simulink model "CubeSatModel_pert"  (R2024a)
settings: Solver=FixedStepAuto  StartTime=0.0  StopTime=5467.6512  FixedStep=0.5  MaxStep=10  RelTol=1e-6  AbsTol=1e-7
undefined symbols (not defined in the file): juliandate
libraries: aerolibutil x12, aerolibconvert2 x4, slpidlib x1, sharedtransform x1, aerolibsatdyn x1, aerolibobsolete x1, aerolibattitudesys x1, simulink x1, vrlib x1
settings Model: Creator=The MathWorks, Inc.  LastModifiedBy=sandr
settings SolverCC: MaxConsecutiveMinStep=10  AutoInsertRateTranBlk=on  DecoupledContinuousIntegration=on  MinimalZcImpactIntegration=on  MaxZcPerStep=1
settings DebuggingCC: ReadBeforeWriteMsg=DisableAll  WriteAfterWriteMsg=DisableAll  WriteAfterReadMsg=DisableAll  MultiTaskDSMMsg=none  UnconnectedInputMsg=warning  UnconnectedOutputMsg=warning  UnconnectedLineMsg=warning
settings ModelReferenceCC: UpdateModelReferenceTargets=IfOutOfDate  EnableRefExpFcnMdlSchedulingChecks=on
settings SFSimCC: SFSimEcho=off
settings RTWCC: GPUComputeCapability=3.5  DLArmComputeVersion=19.05

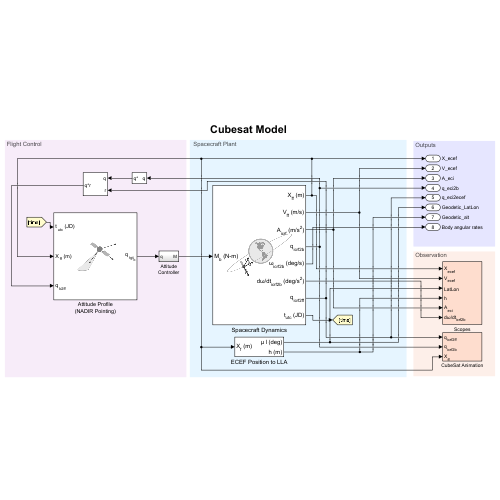
[thumbnail: Simulink's stored preview of the top-level diagram]
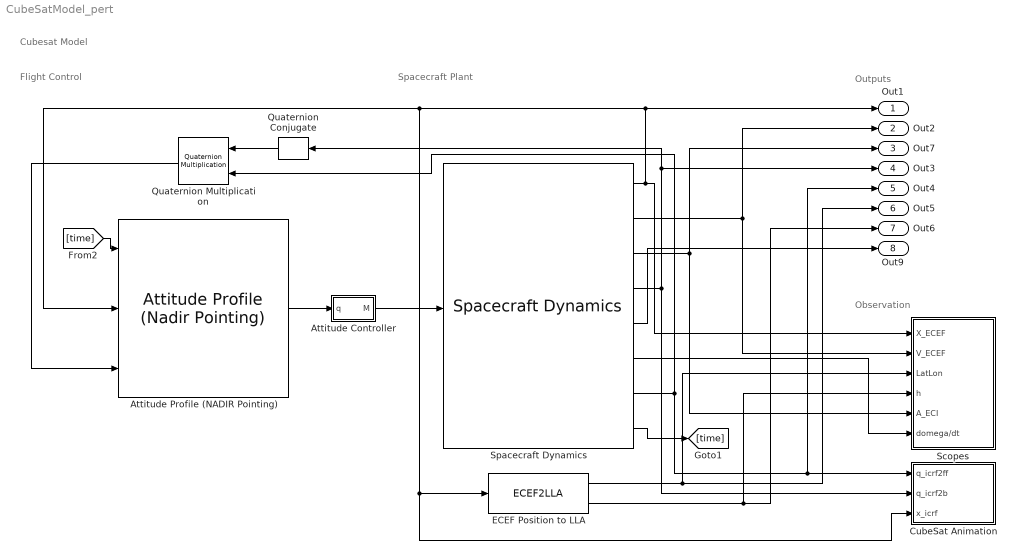
== system CubeSatModel_pert ==
  note: Flight Control
  note: Outputs
  note: Spacecraft Plant
  note: Observation
  note: Cubesat Model
  Attitude Controller : Subsystem
  Attitude Profile (NADIR Pointing) : aerolibsatdyn/Attitude Profile (Nadir Pointing)  outputError=on  outputFinalAttitude=off  portFrame=Fixed-frame  pointingMode=Point at nadir  celestialTarget=Sun  tunablePointing=off  primaryAlignmentSrc=Dialog  primaryAlignment=[0 0 1]  secondaryAlignmentSrc=Dialog  secondaryAlignment=[1 0 0]  constraintFrame=ICRF  primaryConstraintSrc=Dialog  primaryConstraint=[1 0 0]  secondaryConstraintSrc=Dialog  secondaryConstraint=[0 1 0]
  CubeSat Animation : Subsystem  mask(Simulink 3D Animation of CubeSat){enableVis=on, startDate=juliandate(2020, 1, 1, 12, 0, 0), visSampleTime=5, cubesatSize=2e5, showAntenna=on, antennaHeight=1e6, antennaHalfAngle=15}
      mask prompts: enableVis "spacecraft:cubesat:AnimEnableVis"; startDate "spacecraft:cubesat:StartDate"; visSampleTime "spacecraft:cubesat:AnimSampleTime"; cubesatSize "spacecraft:cubesat:MdlSize"; showAntenna "spacecraft:cubesat:ShowCone"; antennaHeight "spacecraft:cubesat:ConeHeight"; antennaHalfAngle "spacecraft:cubesat:ConeAngle"
      mask help: spacecraft:cubesat:VisBlockDesc
      settings: OpenFcn=|
      | if ~builtin('license','test','virtual_reality_toolbox')
      |     set_param(gcb, 'enableVis', 'off');
      | end
      | open_system(gcb,'mask');
      mask Callback enableVis:
      | if strcmp(get_param(gcb,'enableVis'), 'on')
      |     [licAvail, ~] = builtin('license','checkout','Virtual_Reality_Toolbox');
      |     if licAvail
      |         enable = repmat({'on'},7,1);
      |         set_param(gcb, 'Commented', 'off');
      |     else
      |         enable = repmat({'off'},7,1);
      |         set_param(gcb, 'Commented', 'on');
      |         set_param(gcb,'enableVis', 'off');
      |     end
      |     clear licAvail
      | else
      |     enable = repmat({'off'},7,1);
      |     set_param(gcb, 'Commented', 'on');
      | end
      | enable{1} = 'on';
      | set_param(gcb,'MaskEnables', enable);
      | clear enable
      mask Callback showAntenna:
      | if strcmp(get_param(gcb, 'enableVis'), 'on')
      |     enable = get_param(gcb,'MaskEnables');
      |     if strcmp(get_param(gcb, 'showAntenna'), 'off')
      |         enable(6:7) = {'off'};
      |     else
      |         enable(6:7) = {'on'};
      |     end
      |     set_param(gcb,'MaskEnables', enable);
      |     clear enable
      | end
      mask DialogControl enableVis Prompt: Enable visualization with Simulink 3D Animation
      mask DialogControl vrOpenBtn Prompt: spacecraft:cubesat:AnimOpenBtn
      mask DialogControl vrOpenBtn Callback:
      | if builtin('license','checkout','Virtual_Reality_Toolbox')
      |     vrmfunc('FnOpen',getSimulinkBlockHandle([gcb '/VR Sink']));
      | end
      mask DialogControl startDate Prompt: Start date [Julian date]:
      mask DialogControl startDate Tooltip: spacecraft:cubesat:StartDateTT
      mask DialogControl visSampleTime Prompt: Animation refresh rate:
      mask DialogControl visSampleTime Tooltip: spacecraft:cubesat:AnimSampleTimeTT
      mask DialogControl cubesatSize Prompt: CubeSat display size [m]:
      mask DialogControl cubesatSize Tooltip: spacecraft:cubesat:MdlSizeTT
      mask DialogControl Container3 Prompt: spacecraft:cubesat:AntennaPropArea
      mask DialogControl showAntenna Prompt: Show antenna cone in animation
      mask DialogControl showAntenna Tooltip: spacecraft:cubesat:ShowConeTT
      mask DialogControl antennaHeight Prompt: Antenna cone height [m]:
      mask DialogControl antennaHeight Tooltip: spacecraft:cubesat:ConeHeightTT
      mask DialogControl antennaHalfAngle Prompt: Antenna cone half angle [deg]:
      mask DialogControl antennaHalfAngle Tooltip: spacecraft:cubesat:ConeAngleTT
      mask Display:
      | port_label('input', 3, 'X_{ff}','texmode','on')
      | port_label('input', 2, 'q_{icrf2b}','texmode','on')
      | port_label('input', 1, 'q_{icrf2ff}','texmode','on')
  ECEF Position to LLA : ECEF2LLA  R=6378137
  Quaternion Conjugate : aerolibutil/Quaternion Conjugate
  Quaternion Multiplication : aerolibutil/Quaternion Multiplication
  Scopes : Subsystem  VariantControl=visOff
      mask Display:
      | port_label('input', 1, 'X_{ecef}','texmode','on')
      | port_label('input', 2, 'V_{ecef}','texmode','on')
      | port_label('input', 3, 'LatLon','texmode','on')
      | port_label('input', 4, 'h','texmode','on')
      | port_label('input', 5, 'A_{eci}','texmode','on')
      | port_label('input', 6, 'dω/dt_{icrf2b}','texmode','on')
  Spacecraft Dynamics : SpacecraftDynamics  forcesIn=off  accelFrame=Fixed-frame  outportFrame=Fixed-frame  outputAccel=on  startDate=2456824  mass=mission.CubeSat.m  inertia=mission.CubeSat.I  semiMajorAxis=mission.CubeSat.SemiMajorAxis  eccentricity=mission.CubeSat.Eccentricity  inclination=mission.CubeSat.Inclination  raan=mission.CubeSat.RAAN  argPeriapsis=mission.CubeSat.ArgOfPeriapsis  trueAnomaly=mission.CubeSat.TrueAnomaly  inertialPosition=[3649700.0 3308200.0 -4676600.0]  inertialVelocity=[-2750.8 6666.4 2573.4]  fixedPosition=[-2750.8 6666.4 2573.4]  fixedVelocity=[1452.7 -6720.7 2568.1]  attitude=[0.5963 -0.1096 -0.4052 0.6842]  outputAngAccel=on  outputTransform=on  useDrag=on  fluxFlags=ones(1,23)  dragArea=mission.CubeSat.A  ephemerisStartDate=juliandate(2010, 1, 1)  ephemerisEndDate=juliandate(2030, 1, 1)  useThirdBodyGravity=on  useSRP=on  srpArea=mission.CubeSat.A
  Out1 : Outport  SignalName=X_ecef
  Out2 : Outport  Port=2  SignalName=V_ecef
  Out7 : Outport  Port=3  SignalName=A_eci
  Out3 : Outport  Port=4  SignalName=q_eci2b
  Out4 : Outport  Port=5  SignalName=q_eci2ecef
  Out5 : Outport  Port=6  SignalName=Geodetic_LatLon
  Out6 : Outport  Port=7  SignalName=Geodetic_alt
  Out9 : Outport  Port=8  SignalName=Body angular rates
  wires:
  Spacecraft Dynamics/2 -> Scopes/2(V_ECEF), Out2/1
  Spacecraft Dynamics/1 -> Scopes/1(X_ECEF), ECEF Position to LLA/1, CubeSat Animation/3(x_icrf), Attitude Profile (NADIR Pointing)/2, Out1/1
  Spacecraft Dynamics/4 -> Out3/1, Quaternion Conjugate/1, CubeSat Animation/2(q_icrf2b)
  Attitude Profile (NADIR Pointing)/1 -> Attitude Controller/1(q)
  Quaternion Multiplication/1 -> Attitude Profile (NADIR Pointing)/3
  Spacecraft Dynamics/3 -> Scopes/5(A_ECI), Out7/1
  Spacecraft Dynamics/5 -> Out9/1
  ECEF Position to LLA/2 -> Scopes/4(h), Out6/1
  Spacecraft Dynamics/7 -> Quaternion Multiplication/2, Out4/1, CubeSat Animation/1(q_icrf2ff)
  Attitude Controller/1(M) -> Spacecraft Dynamics/1
  ECEF Position to LLA/1 -> Scopes/3(LatLon), Out5/1
  Spacecraft Dynamics/8 -> [time]
  [time] -> Attitude Profile (NADIR Pointing)/1
  Quaternion Conjugate/1 -> Quaternion Multiplication/1
  Spacecraft Dynamics/6 -> Scopes/6(domega/dt)

== system CubeSatModel_pert/Attitude Controller ==
  q : Inport
  Demo Controller : slpidlib/PID Controller  Controller=PD  Form=Parallel  TimeDomain=Discrete-time  UseExternalTs=off  SampleTime=-1  IntegratorMethod=Trapezoidal  FilterMethod=Trapezoidal  ControllerParametersSource=internal  P=.000055  I=0  UseKiTs=off  D=.017  UseExternalDerivativeSource=off  N=1  UseFilter=off  TunerSelectOption=Transfer Function Based (PID Tuner App)  InitialConditionSource=internal  InitialConditionForIntegrator=0  InitialConditionForFilter=0  DifferentiatorICPrevScaledInput=0  ExternalReset=none  TrackingMode=off  Kt=1  LimitOutput=on  SatLimitsSource=internal  UpperSaturationLimit=0.008  LowerSaturationLimit=-0.008  LinearizeAsGain=on  AntiWindupMode=none  Kb=1  LimitIntegrator=off  UpperIntegratorSaturationLimit=inf  LowerIntegratorSaturationLimit=-inf  POutMin=[]  POutMax=[]  IOutMin=[]  IOutMax=[]  DOutMin=[]  DOutMax=[]  NOutMin=[]  NOutMax=[]  SumOutMin=[]  SumOutMax=[]  SaturationOutMin=[]  SaturationOutMax=[]  PParamMin=[]  PParamMax=[]  IParamMin=[]  IParamMax=[]  DParamMin=[]  DParamMax=[]  NParamMin=[]  NParamMax=[]  KbParamMin=[]  KbParamMax=[]  KtParamMin=[]  KtParamMax=[]  KbOutMin=[]  KbOutMax=[]  KtOutMin=[]  KtOutMax=[]  IntegratorOutMin=[]  IntegratorOutMax=[]  FilterOutMin=[]  FilterOutMax=[]  SumI1OutMin=[]  SumI1OutMax=[]  SumI2OutMin=[]  SumI2OutMax=[]  SumI3OutMin=[]  SumI3OutMax=[]  SumI4OutMin=[]  SumI4OutMax=[]  SumDOutMin=[]  SumDOutMax=[]  DifferentiatorOutMin=[]  DifferentiatorOutMax=[]  FilterDiffOutCoefMin=[]  FilterDiffOutCoefMax=[]  ReciprocalOutMin=[]  ReciprocalOutMax=[]  SumDenOutMin=[]  SumDenOutMax=[]  SumNumOutMin=[]  SumNumOutMax=[]  DivideOutMin=[]  DivideOutMax=[]  UdiffTsProdOutMin=[]  UdiffTsProdOutMax=[]  NTsProdOutMin=[]  NTsProdOutMax=[]  UintegralTsProdOutMin=[]  UintegralTsProdOutMax=[]  UngainTsProdOutMin=[]  UngainTsProdOutMax=[]  ClampingZeroOutDataTypeStr=Inherit: Inherit via back propagation  ClampingZeroOutMin=[]  ClampingZeroOutMax=[]  FilterDenConstantOutDataTypeStr=Inherit: Inherit via back propagation  FilterDenConstantOutMin=[]  FilterDenConstantOutMax=[]  PCopyOutDataTypeStr=Inherit: Inherit via back propagation  PCopyOutMin=[]  PCopyOutMax=[]  NCopyOutDataTypeStr=Inherit: Inherit via back propagation  NCopyOutMin=[]  NCopyOutMax=[]  IntegratorContinuousStateAttributes=''  IntegratorStateMustResolveToSignalObject=off  IntegratorRTWStateStorageClass=Auto  FilterContinuousStateAttributes=''  FilterStateMustResolveToSignalObject=off  FilterRTWStateStorageClass=Auto  ParallelPVariant=InternalParameters  IdealPVariant=Disabled  IVariant=Disabled  DVariant=InternalParameters  IntegratorVariant=Disabled  SatVariant=Enabled  AWVariant=Disabled  PCopyVariant=Disabled  TRVariant=Disabled  FdbkBlocksVariant=Forward  IdealPFdbkVariant=Disabled  SatFdbkVariant=Disabled  DerivativeFilterVariant=Differentiator  NVariant=Passthrough  NCopyVariant=Disabled_SignalSpec  FilterICVariant=InternalICsDifferentiator  IntegratorICVariant=Disabled  ExternalResetVariant=Disabled  TRSumVariant=Passthrough  SumFdbkVariant=Disabled  SumVariant=Sum_PD  TsampFilterVariant=InternalTs  TsampNgainVariant=Passthrough  TsampIntegralVariant=Disabled_SignalSpec  ExternalSaturationOutDataTypeStr=Inherit: Same as second input  DerivativeSourceVariant=ErrorSignal
  Quaternions to Rotation Angles : sharedtransform/Quaternions to Rotation Angles  rotationOrder=XYZ  aMode=aMode
  M : Outport
  wires:
  q/1 -> Quaternions to Rotation Angles/1
  Quaternions to Rotation Angles/1 -> Demo Controller/1
  Demo Controller/1 -> M/1

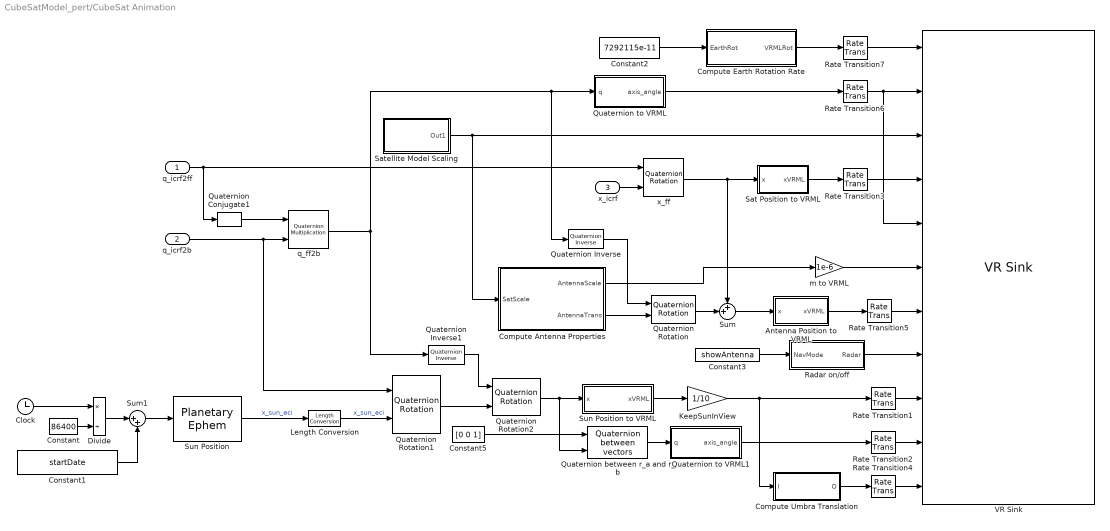
== system CubeSatModel_pert/CubeSat Animation ==
  q_icrf2ff : Inport  PortDimensions=4
  q_icrf2b : Inport  Port=2  PortDimensions=4
  x_icrf : Inport  Port=3  PortDimensions=3
  Antenna Position to VRML : Subsystem
  Clock : Clock
  Compute Antenna Properties : Subsystem
  Compute Earth Rotation Rate : Subsystem
  Compute Umbra Translation : Subsystem
  Constant : Constant  Value=86400
  Constant1 : Constant  Value=startDate  SampleTime=visSampleTime
  Constant2 : Constant  Value=7292115e-11
  Constant3 : Constant  Value=showAntenna
  Constant5 : Constant  Value=[0 0 1]
  Divide : Product  Inputs=*/
  KeepSunInView : Gain  Gain=1/10
  Length Conversion : aerolibconvert2/Length Conversion  IU=km  OU=m
  Quaternion Conjugate1 : aerolibutil/Quaternion Conjugate
  Quaternion Inverse : aerolibutil/Quaternion Inverse
  Quaternion Inverse1 : aerolibutil/Quaternion Inverse
  Quaternion Rotation : aerolibutil/Quaternion Rotation
  Quaternion Rotation1 : aerolibutil/Quaternion Rotation
  Quaternion Rotation2 : aerolibutil/Quaternion Rotation
  Quaternion between r_a and r_b : aerolibattitudesys/Quaternion between vectors
  Quaternion to VRML : Subsystem
  Quaternion to VRML1 : Subsystem
  Radar on/off : Subsystem
  Rate Transition{1..7} (7 alike) : RateTransition
  Sat Position to VRML : Subsystem
  Satellite Model Scaling : Subsystem
  Sum : Sum  Inputs=++|
  Sum1 : Sum  Inputs=|++
  Sun Position : PlanetaryEphem  ephemerisModel=DE421  target=Sun  outputVelocity=off
  Sun Position to VRML : Subsystem
  VR Sink : vrlib/VR Sink  InstantiateOnLoad=on  SampleTime=visSampleTime  ViewEnable=on  RemoteChange=off  RemoteView=off  FieldsWritten=Earth.rotation.4.1.1.double#Satellite.rotation.4.1.1.double#Satellite.scale.3.1.1.double#Satellite.translation.3.1.1.double#AntennaCone.rotation.4.1.1.double#AntennaCone.scale.3.1.1.double#AntennaCone.translation.3.1.1.double#AntennaMaterial.transparency.1.1.1.double#Sun.translation.3.1.1.double#Umbra.rotation.4.1.1.double#Umbra.translation.3.1.1.double  WorldFileName=cubesatAnim.wrl  WorldDescription=CubeSat Orbit Animation  AutoView=off  VideoDimensions=[]  AllowVariableSize=off
  m to VRML : Gain  Gain=1e-6
  q_ff2b : aerolibutil/Quaternion Multiplication
  x_ff : aerolibutil/Quaternion Rotation
  wires:
  Quaternion to VRML1/1(axis_angle) -> Rate Transition2/1
  Quaternion between r_a and r_b/1 -> Quaternion to VRML1/1(q)
  Constant2/1 -> Compute Earth Rotation Rate/1(EarthRot)
  Compute Antenna Properties/1(AntennaScale) -> m to VRML/1
  Quaternion to VRML/1(axis_angle) -> Rate Transition6/1
  Compute Umbra Translation/1(O) -> Rate Transition4/1
  q_icrf2b/1 -> Quaternion Rotation1/1, q_ff2b/2
  Quaternion Rotation2/1 -> Sun Position to VRML/1(x), Quaternion between r_a and r_b/2
  Constant5/1 -> Quaternion between r_a and r_b/1
  KeepSunInView/1 -> Compute Umbra Translation/1(I), Rate Transition1/1
  Sun Position to VRML/1(xVRML) -> KeepSunInView/1
  Sat Position to VRML/1(xVRML) -> Rate Transition3/1
  Compute Antenna Properties/2(AntennaTrans) -> Quaternion Rotation/2
  Satellite Model Scaling/1(Out1) -> VR Sink/3, Compute Antenna Properties/1(SatScale)
  Constant3/1 -> Radar on/off/1(NavMode)
  q_ff2b/1 -> Quaternion Inverse/1, Quaternion to VRML/1(q), Quaternion Inverse1/1
  Quaternion Rotation1/1 -> Quaternion Rotation2/2
  Compute Earth Rotation Rate/1(VRMLRot) -> Rate Transition7/1
  Antenna Position to VRML/1(xVRML) -> Rate Transition5/1
  Quaternion Inverse/1 -> Quaternion Rotation/1
  x_ff/1 -> Sum/1, Sat Position to VRML/1(x)
  Quaternion Rotation/1 -> Sum/2
  Sum/1 -> Antenna Position to VRML/1(x)
  Quaternion Inverse1/1 -> Quaternion Rotation2/1
  Rate Transition4/1 -> VR Sink/11
  Rate Transition2/1 -> VR Sink/10
  Rate Transition1/1 -> VR Sink/9
  Rate Transition5/1 -> VR Sink/7
  m to VRML/1 -> VR Sink/6
  Rate Transition3/1 -> VR Sink/4
  Rate Transition7/1 -> VR Sink/1
  Rate Transition6/1 -> VR Sink/5, VR Sink/2
  Constant1/1 -> Sum1/2
  Divide/1 -> Sum1/1
  Constant/1 -> Divide/2
  Sun Position/1 -> Length Conversion/1  "x_sun_eci"
  Clock/1 -> Divide/1
  Length Conversion/1 -> Quaternion Rotation1/2  "x_sun_eci"
  Sum1/1 -> Sun Position/1
  Radar on/off/1(Radar) -> VR Sink/8
  Quaternion Conjugate1/1 -> q_ff2b/1
  q_icrf2ff/1 -> Quaternion Conjugate1/1, x_ff/1
  x_icrf/1 -> x_ff/2

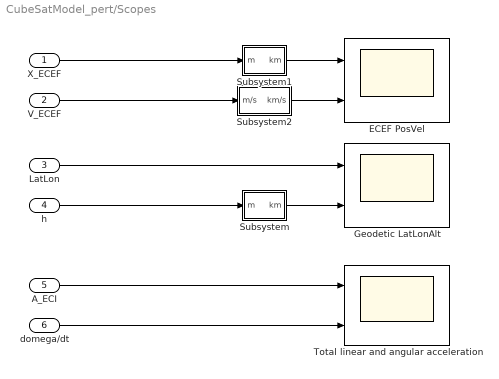
== system CubeSatModel_pert/Scopes ==
  X_ECEF : Inport
  V_ECEF : Inport  Port=2
  LatLon : Inport  Port=3
  h : Inport  Port=4
  A_ECI : Inport  Port=5
  domega/dt : Inport  Port=6
  ECEF PosVel : Scope  NumInputPorts=2
  Geodetic LatLonAlt : Scope  NumInputPorts=2
  Subsystem : Subsystem
  Subsystem1 : Subsystem
  Subsystem2 : Subsystem
  Total linear and angular acceleration : Scope  NumInputPorts=2
  wires:
  V_ECEF/1 -> Subsystem2/1(m/s)
  X_ECEF/1 -> Subsystem1/1(m)
  Subsystem/1(km) -> Geodetic LatLonAlt/2
  Subsystem1/1(km) -> ECEF PosVel/1
  Subsystem2/1(km/s) -> ECEF PosVel/2
  h/1 -> Subsystem/1(m)
  LatLon/1 -> Geodetic LatLonAlt/1
  A_ECI/1 -> Total linear and angular acceleration/1
  domega/dt/1 -> Total linear and angular acceleration/2

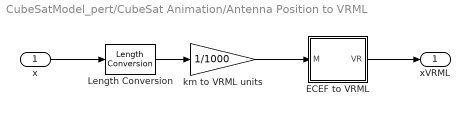
== system CubeSatModel_pert/CubeSat Animation/Antenna Position to VRML ==
  x : Inport
  ECEF to VRML : Subsystem
  Length Conversion : aerolibconvert2/Length Conversion  IU=m  OU=km
  km to VRML units : Gain  Gain=1/1000
  xVRML : Outport  VectorParamsAs1DForOutWhenUnconnected=off
  wires:
  Length Conversion/1 -> km to VRML units/1
  km to VRML units/1 -> ECEF to VRML/1(M)
  x/1 -> Length Conversion/1
  ECEF to VRML/1(VR) -> xVRML/1

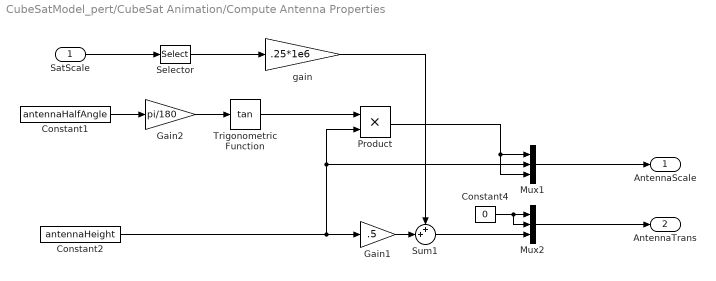
== system CubeSatModel_pert/CubeSat Animation/Compute Antenna Properties ==
  SatScale : Inport
  Constant1 : Constant  Value=antennaHalfAngle
  Constant2 : Constant  Value=antennaHeight
  Constant4 : Constant  Value=0
  Gain1 : Gain  Gain=.5
  Gain2 : Gain  Gain=pi/180
  Mux1 : Mux  Inputs=3
  Mux2 : Mux  Inputs=3
  Product : Product
  Selector : Selector  InputPortWidth=3  IndexOptions=Index vector (dialog)  Indices=1  OutputSizes=1
  Sum1 : Sum  Inputs=++|
  Trigonometric Function : Trigonometry  Operator=tan
  gain : Gain  Gain=.25*1e6
  AntennaScale : Outport  VectorParamsAs1DForOutWhenUnconnected=off
  AntennaTrans : Outport  Port=2  VectorParamsAs1DForOutWhenUnconnected=off
  wires:
  Gain2/1 -> Trigonometric Function/1
  Constant4/1 -> Mux2/1, Mux2/2
  Sum1/1 -> Mux2/3
  Constant2/1 -> Gain1/1, Mux1/2, Product/2
  gain/1 -> Sum1/1
  Constant1/1 -> Gain2/1
  Product/1 -> Mux1/3, Mux1/1
  Gain1/1 -> Sum1/2
  Trigonometric Function/1 -> Product/1
  Mux2/1 -> AntennaTrans/1
  Mux1/1 -> AntennaScale/1
  SatScale/1 -> Selector/1
  Selector/1 -> gain/1

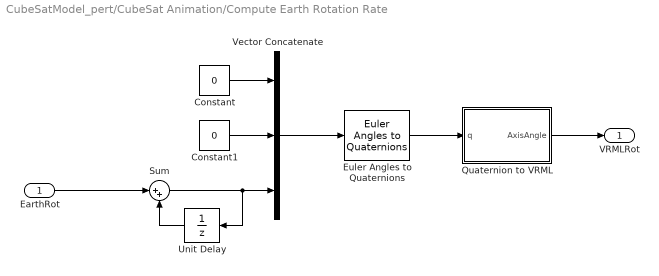
== system CubeSatModel_pert/CubeSat Animation/Compute Earth Rotation Rate ==
  EarthRot : Inport
  Constant : Constant  Value=0
  Constant1 : Constant  Value=0
  Euler Angles to Quaternions : aerolibobsolete/Euler Angles to Quaternions
  Quaternion to VRML : Subsystem
  Sum : Sum  Inputs=|++
  Unit Delay : UnitDelay  SampleTime=-1  HasFrameUpgradeWarning=on
  Vector Concatenate : Concatenate  NumInputs=3
  VRMLRot : Outport  VectorParamsAs1DForOutWhenUnconnected=off
  wires:
  Quaternion to VRML/1(AxisAngle) -> VRMLRot/1
  Euler Angles to Quaternions/1 -> Quaternion to VRML/1(q)
  Vector Concatenate/1 -> Euler Angles to Quaternions/1
  Constant1/1 -> Vector Concatenate/2
  Constant/1 -> Vector Concatenate/1
  Sum/1 -> Unit Delay/1, Vector Concatenate/3
  Unit Delay/1 -> Sum/2
  EarthRot/1 -> Sum/1

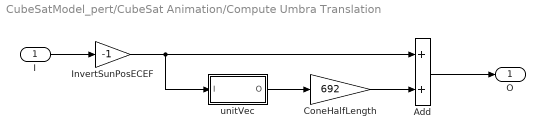
== system CubeSatModel_pert/CubeSat Animation/Compute Umbra Translation ==
  I : Inport
  Add : Sum
  ConeHalfLength : Gain  Gain=692
  InvertSunPosECEF : Gain  Gain=-1
  unitVec : Subsystem
  O : Outport  VectorParamsAs1DForOutWhenUnconnected=off
  wires:
  ConeHalfLength/1 -> Add/2
  I/1 -> InvertSunPosECEF/1
  Add/1 -> O/1
  InvertSunPosECEF/1 -> unitVec/1(I), Add/1
  unitVec/1(O) -> ConeHalfLength/1

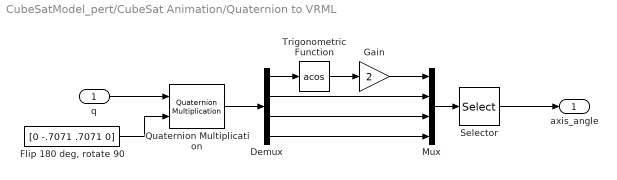
== system CubeSatModel_pert/CubeSat Animation/Quaternion to VRML ==
  q : Inport
  Demux : Demux
  "Flip 180 deg, rotate 90" : Constant  Value=[0 -.7071 .7071 0]
  Gain : Gain  Gain=2
  Mux : Mux
  Quaternion Multiplication : aerolibutil/Quaternion Multiplication
  Selector : Selector  InputPortWidth=4  IndexOptions=Index vector (dialog)  Indices=[3 4 2 1]  OutputSizes=1
  Trigonometric Function : Trigonometry  Operator=acos
  axis_angle : Outport  VectorParamsAs1DForOutWhenUnconnected=off
  wires:
  Demux/4 -> Mux/4
  Demux/3 -> Mux/3
  Demux/2 -> Mux/2
  Gain/1 -> Mux/1
  Selector/1 -> axis_angle/1
  q/1 -> Quaternion Multiplication/1
  Mux/1 -> Selector/1
  Trigonometric Function/1 -> Gain/1
  Demux/1 -> Trigonometric Function/1
  "Flip 180 deg, rotate 90"/1 -> Quaternion Multiplication/2
  Quaternion Multiplication/1 -> Demux/1

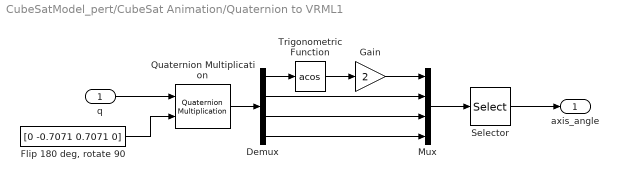
== system CubeSatModel_pert/CubeSat Animation/Quaternion to VRML1 ==
  q : Inport
  Demux : Demux
  "Flip 180 deg, rotate 90" : Constant  Value=[0 -0.7071 0.7071 0]
  Gain : Gain  Gain=2
  Mux : Mux
  Quaternion Multiplication : aerolibutil/Quaternion Multiplication
  Selector : Selector  InputPortWidth=4  IndexOptions=Index vector (dialog)  Indices=[3 4 2 1]  OutputSizes=1
  Trigonometric Function : Trigonometry  Operator=acos
  axis_angle : Outport  VectorParamsAs1DForOutWhenUnconnected=off
  wires:
  Demux/4 -> Mux/4
  Demux/3 -> Mux/3
  Demux/2 -> Mux/2
  Gain/1 -> Mux/1
  Selector/1 -> axis_angle/1
  Mux/1 -> Selector/1
  Trigonometric Function/1 -> Gain/1
  Demux/1 -> Trigonometric Function/1
  "Flip 180 deg, rotate 90"/1 -> Quaternion Multiplication/2
  q/1 -> Quaternion Multiplication/1
  Quaternion Multiplication/1 -> Demux/1

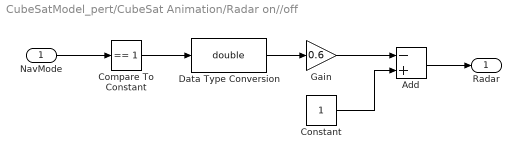
== system CubeSatModel_pert/CubeSat Animation/Radar on//off ==
  NavMode : Inport
  Add : Sum  Inputs=-+
  Compare To Constant : simulink/Logic and Bit Operations/Compare To Constant  relop===  const=1  OutDataTypeStr=boolean  ZeroCross=off
  Constant : Constant
  Data Type Conversion : DataTypeConversion  OutDataTypeStr=double  SaturateOnIntegerOverflow=off  RndMeth=Floor
  Gain : Gain  Gain=0.6
  Radar : Outport  VectorParamsAs1DForOutWhenUnconnected=off
  wires:
  NavMode/1 -> Compare To Constant/1
  Compare To Constant/1 -> Data Type Conversion/1
  Data Type Conversion/1 -> Gain/1
  Gain/1 -> Add/1
  Constant/1 -> Add/2
  Add/1 -> Radar/1

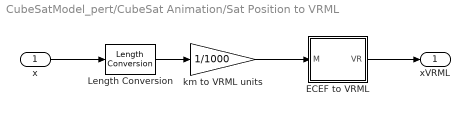
== system CubeSatModel_pert/CubeSat Animation/Sat Position to VRML ==
  x : Inport
  ECEF to VRML : Subsystem
  Length Conversion : aerolibconvert2/Length Conversion  IU=m  OU=km
  km to VRML units : Gain  Gain=1/1000
  xVRML : Outport  VectorParamsAs1DForOutWhenUnconnected=off
  wires:
  ECEF to VRML/1(VR) -> xVRML/1
  x/1 -> Length Conversion/1
  km to VRML units/1 -> ECEF to VRML/1(M)
  Length Conversion/1 -> km to VRML units/1

== system CubeSatModel_pert/CubeSat Animation/Satellite Model Scaling ==
  Constant : Constant  Value=cubesatSize
  Mux : Mux  Inputs=3
  ScaleModelToVRML : Gain  Gain=1/.3e6
  Out1 : Outport  VectorParamsAs1DForOutWhenUnconnected=off
  wires:
  ScaleModelToVRML/1 -> Mux/3, Mux/1, Mux/2
  Constant/1 -> ScaleModelToVRML/1
  Mux/1 -> Out1/1

== system CubeSatModel_pert/CubeSat Animation/Sun Position to VRML ==
  x : Inport
  ECEF to VRML : Subsystem
  Length Conversion : aerolibconvert2/Length Conversion  IU=m  OU=km
  km to VRML units : Gain  Gain=1/1000
  xVRML : Outport  VectorParamsAs1DForOutWhenUnconnected=off
  wires:
  ECEF to VRML/1(VR) -> xVRML/1
  x/1 -> Length Conversion/1
  km to VRML units/1 -> ECEF to VRML/1(M)
  Length Conversion/1 -> km to VRML units/1

== system CubeSatModel_pert/Scopes/Subsystem ==
  m : Inport  Unit=m
  Unit Conversion : UnitConversion
  km : Outport  Unit=km  VectorParamsAs1DForOutWhenUnconnected=off
  wires:
  Unit Conversion/1 -> km/1
  m/1 -> Unit Conversion/1

== system CubeSatModel_pert/Scopes/Subsystem1 ==
  m : Inport  Unit=m
  Unit Conversion : UnitConversion
  km : Outport  Unit=km  VectorParamsAs1DForOutWhenUnconnected=off
  wires:
  m/1 -> Unit Conversion/1
  Unit Conversion/1 -> km/1

== system CubeSatModel_pert/Scopes/Subsystem2 ==
  m/s : Inport  Unit=m/s
  Unit Conversion : UnitConversion
  km/s : Outport  Unit=km/s  VectorParamsAs1DForOutWhenUnconnected=off
  wires:
  Unit Conversion/1 -> km/s/1
  m/s/1 -> Unit Conversion/1

== system CubeSatModel_pert/CubeSat Animation/Antenna Position to VRML/ECEF to VRML ==
  M : Inport  PortDimensions=3
  Selector : Selector  InputPortWidth=3  IndexOptions=Index vector (dialog)  Indices=[2 3 1]  OutputSizes=1
  VR : Outport  PortDimensions=3  VectorParamsAs1DForOutWhenUnconnected=off
  wires:
  M/1 -> Selector/1
  Selector/1 -> VR/1

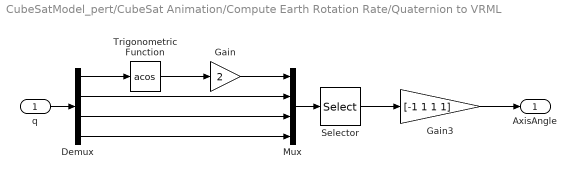
== system CubeSatModel_pert/CubeSat Animation/Compute Earth Rotation Rate/Quaternion to VRML ==
  q : Inport
  Demux : Demux
  Gain : Gain  Gain=2
  Gain3 : Gain  Gain=[-1 1 1 1]
  Mux : Mux
  Selector : Selector  InputPortWidth=4  IndexOptions=Index vector (dialog)  Indices=[2 4 3 1]  OutputSizes=1
  Trigonometric Function : Trigonometry  Operator=acos
  AxisAngle : Outport  VectorParamsAs1DForOutWhenUnconnected=off
  wires:
  Demux/1 -> Trigonometric Function/1
  Trigonometric Function/1 -> Gain/1
  Mux/1 -> Selector/1
  q/1 -> Demux/1
  Gain3/1 -> AxisAngle/1
  Selector/1 -> Gain3/1
  Gain/1 -> Mux/1
  Demux/2 -> Mux/2
  Demux/3 -> Mux/3
  Demux/4 -> Mux/4

== system CubeSatModel_pert/CubeSat Animation/Compute Umbra Translation/unitVec ==
  I : Inport
  Divide : Product  Inputs=*/
  Dot Product : DotProduct  OutDataTypeStr=Inherit: Inherit via internal rule
  Sqrt : Sqrt
  O : Outport  VectorParamsAs1DForOutWhenUnconnected=off
  wires:
  Dot Product/1 -> Sqrt/1
  I/1 -> Divide/1, Dot Product/1, Dot Product/2
  Divide/1 -> O/1
  Sqrt/1 -> Divide/2

== system CubeSatModel_pert/CubeSat Animation/Sat Position to VRML/ECEF to VRML ==
  M : Inport  PortDimensions=3
  Selector : Selector  InputPortWidth=3  IndexOptions=Index vector (dialog)  Indices=[2 3 1]  OutputSizes=1
  VR : Outport  PortDimensions=3  VectorParamsAs1DForOutWhenUnconnected=off
  wires:
  M/1 -> Selector/1
  Selector/1 -> VR/1

== system CubeSatModel_pert/CubeSat Animation/Sun Position to VRML/ECEF to VRML ==
  M : Inport  PortDimensions=3
  Selector : Selector  InputPortWidth=3  IndexOptions=Index vector (dialog)  Indices=[2 3 1]  OutputSizes=1
  VR : Outport  PortDimensions=3  VectorParamsAs1DForOutWhenUnconnected=off
  wires:
  M/1 -> Selector/1
  Selector/1 -> VR/1
